simulink model "luenberger_generatedata"  (R2019b)
settings: Solver=ode45  StartTime=0.0  StopTime=tfinal  MaxStep=.01  RelTol=1e-3  EnableMultiTasking=on
values from neighbouring files (symbols this model uses):
  amp1 = 2    [proofmass_init.m]
  Aobc = [ A,  -B*K; L*C , A-B*K-L*C]    [proofmass_init.m]
  Bobc = [B;B]    [proofmass_init.m]
  Cobc = [C , zeros(size(C)); zeros(size(C)), C]    [proofmass_init.m]
  Dobc = zeros(m,p)    [proofmass_init.m]
  w1 = pi    (= 3.14159265359)    [proofmass_init.m]
  x0_obc = [randn(n/2,1); zeros(n/2,1)]    [proofmass_init.m]
libraries: simulink x1
settings Model: Creator=boswkenn  LastModifiedBy=Shishir
settings DataIOCC: LimitDataPoints=on  SaveFormat=Array  ReturnWorkspaceOutputs=off
settings OptimizationCC: LifeSpan=inf
settings DebuggingCC: UnderspecifiedInitializationDetection=Classic  MergeDetectMultiDrivingBlocksExec=none  SolverPrmCheckMsg=warning  SFUnexpectedBacktrackingDiag=warning  SFNoUnconditionalDefaultTransitionDiag=warning  SFExecutionAtInitializationDiag=none  ArithmeticOperatorsInVariantConditions=warning
settings HardwareCC: ProdBitPerPointer=32  ProdBitPerSizeT=32  ProdBitPerPtrDiffT=32  ProdLargestAtomicFloat=None  ProdIntDivRoundTo=Undefined  ProdEndianess=Unspecified  ProdWordSize=32  ProdHWDeviceType=32-bit Generic
settings ModelReferenceCC: PropagateSignalLabelsOutOfModel=off
settings SFSimCC: SimUseLocalCustomCode=off  CustomCodeUndefinedFunction=UseInterfaceOnly
settings RTWCC: RTWUseLocalCustomCode=off
settings CodeAppCC: StateflowObjectComments=on
settings GRTTargetCC: TargetLangStandard=C89/C90 (ANSI)  GeneratePreprocessorConditionals=Disable all
settings ConfigComp: CovMetricSettings=dw  CovHtmlReporting=on  CovSaveCumulativeToWorkspaceVar=on  CovSaveSingleToWorkspaceVar=on  CovExternalEMLEnable=off

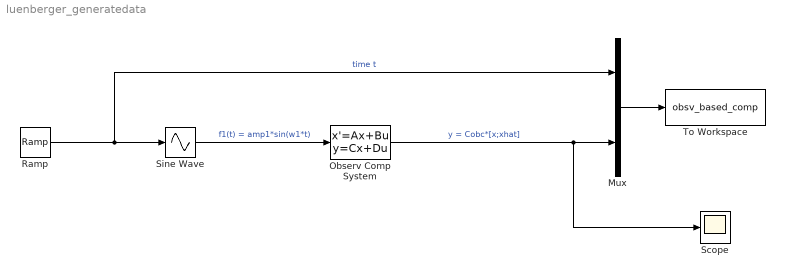
== system luenberger_generatedata ==
  Mux : Mux  Inputs=2
  Observ Comp System : StateSpace  A=Aobc  B=Bobc  C=Cobc  D=Dobc  InitialCondition=x0_obc
  Ramp : simulink/Sources/Ramp  slope=1  start=0  InitialOutput=0
  Scope : Scope
  Sine Wave : Sin  TimeSource=Use external signal  Amplitude=amp1  Frequency=w1  SampleTime=0
  To Workspace : ToWorkspace  VariableName=obsv_based_comp  SampleTime=-1
  wires:
  Observ Comp System/1 -> Scope/1, Mux/2  "y = Cobc*[x;xhat]"
  Ramp/1 -> Mux/1, Sine Wave/1  "time t"
  Mux/1 -> To Workspace/1
  Sine Wave/1 -> Observ Comp System/1  "f1(t) = amp1*sin(w1*t)"
